simulink model "rwdEV_test01"  (R2024a)
settings: Solver=ode23t  StartTime=0.0  StopTime=2  RelTol=1e-3
model workspace (MAT data in the model file):
  f_aud = 100
libraries: fl_lib x9, sdl_lib x7, nesl_utility x6, dspsnks4 x1, ee_lib x1
settings Model: PacingRate=71  Creator=user  LastModifiedBy=user

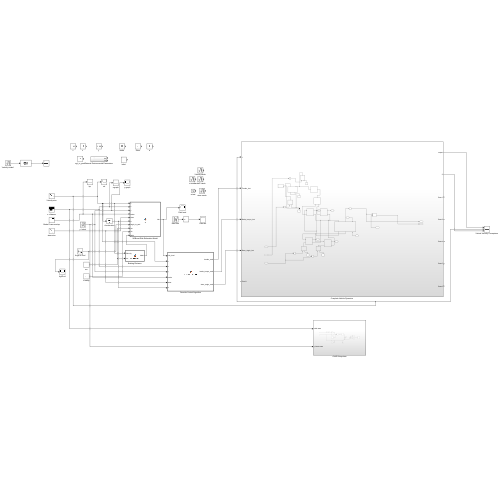
[thumbnail: Simulink's stored preview of the top-level diagram]
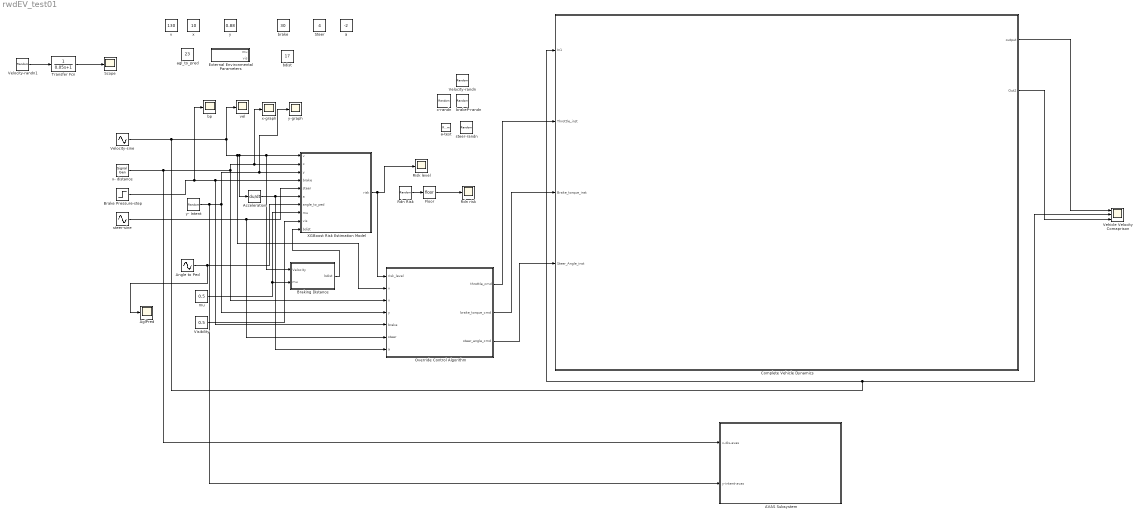
== system rwdEV_test01 ==
  AVAS Subsystem : Subsystem
  Acceleration : Derivative
  AglPred : Scope
  Angle to Ped : Sin  Amplitude=3  Frequency=0.15  SampleTime=0
  Brake Pressure-step : Step  Time=4  Before=0.2  After=0.6  SampleTime=0
  Braking Distance : MATLAB Function  TreatAsAtomicUnit=on
  "Complete Vehicle Dynamics " : Subsystem
  External Environmental Parameters : Subsystem
  Floor : Rounding
  Override Control Algorithm : MATLAB Function  TreatAsAtomicUnit=on
  Rdn Risk : UniformRandomNumber  Minimum=0  Maximum=3  SampleTime=1
  Rdn risk : Scope
  Risk level : Scope
  Scope : Scope
  Steer : Constant  Value=4
  Transfer Fcn : TransferFcn  Denominator=[0.05 1]
  Vehicle Velocity Comaprison : Scope  NumInputPorts=3
  Velocity-randn : RandomNumber  Mean=10  Variance=6  SampleTime=0.1
  Velocity-randn1 : RandomNumber  Mean=10  Variance=6  SampleTime=0.1
  Velocity-sine : Sin  Amplitude=30  Bias=180  Frequency=0.05  SampleTime=0
  Visibility : Constant  Value=0.5
  XGBoost Risk Estimation Model : MATLAB Function  TreatAsAtomicUnit=on
  a : Constant  Value=-2
  a-test : RandomNumber  Mean=3  Variance=2  SampleTime=0.1
  agl_to_pred : Constant  Value=23
  bdist : Constant  Value=17
  bp : Scope
  brake : Constant  Value=30
  brakeP-randn : RandomNumber  Mean=500  Variance=400  SampleTime=0.1
  mu : Constant  Value=0.5
  steer-randn : RandomNumber  Variance=15  SampleTime=0.1
  steer-sine : Sin  Amplitude=2  Bias=5  Frequency=0.2  SampleTime=0
  v : Constant  Value=130
  vel : Scope
  x : Constant  Value=10
  x- distance : SignalGenerator  WaveForm=random  Amplitude=0.1  Frequency=0.3  Units=rad/sec
  x-graph : Scope
  x-randn : RandomNumber  Mean=12  Variance=15  SampleTime=0.1
  y : Constant  Value=0.88
  y- Intent : RandomNumber  Mean=0.2  Variance=0.01  Seed=42  SampleTime=0.1
  y-graph : Scope
  wires:
  XGBoost Risk Estimation Model/1(risk) -> Risk level/1, Override Control Algorithm/1(risk_level)
  y- Intent/1 -> AVAS Subsystem/2(y-intent-avas), y-graph/1, XGBoost Risk Estimation Model/3(y), Override Control Algorithm/4(y)
  mu/1 -> Braking Distance/2(mu), XGBoost Risk Estimation Model/8(mu)
  Visibility/1 -> XGBoost Risk Estimation Model/9(vis)
  Braking Distance/1(bdist) -> XGBoost Risk Estimation Model/10(bdist)
  Angle to Ped/1 -> AglPred/1, XGBoost Risk Estimation Model/7(angle_to_ped)
  Velocity-sine/1 -> Vehicle Velocity Comaprison/2, "Complete Vehicle Dynamics "/1(In1), Override Control Algorithm/2(v), Braking Distance/1(Velocity), XGBoost Risk Estimation Model/1(v), Acceleration/1, vel/1
  x- distance/1 -> AVAS Subsystem/1(x-dis-avas), x-graph/1, XGBoost Risk Estimation Model/2(x), Override Control Algorithm/3(x)
  Brake Pressure-step/1 -> Override Control Algorithm/5(brake), XGBoost Risk Estimation Model/4(brake), bp/1
  steer-sine/1 -> Override Control Algorithm/6(steer), XGBoost Risk Estimation Model/5(steer)
  Acceleration/1 -> Override Control Algorithm/7(a), XGBoost Risk Estimation Model/6(a)
  Velocity-randn1/1 -> Transfer Fcn/1
  Transfer Fcn/1 -> Scope/1
  Rdn Risk/1 -> Floor/1
  Floor/1 -> Rdn risk/1
  Override Control Algorithm/1(throttle_cmd) -> "Complete Vehicle Dynamics "/2(Throttle_inst)
  Override Control Algorithm/2(brake_torque_cmd) -> "Complete Vehicle Dynamics "/3(Brake_torque_inst)
  Override Control Algorithm/3(steer_angle_cmd) -> "Complete Vehicle Dynamics "/4(Steer_Angle_inst)
  "Complete Vehicle Dynamics "/1(output) -> Vehicle Velocity Comaprison/1
  "Complete Vehicle Dynamics "/2(Out2) -> Vehicle Velocity Comaprison/3

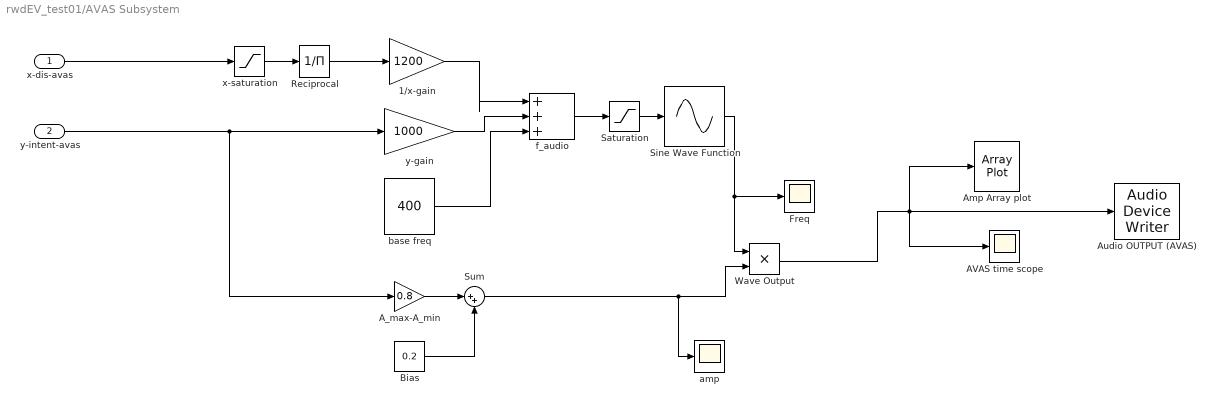
== system rwdEV_test01/AVAS Subsystem ==
  x-dis-avas : Inport
  y-intent-avas : Inport  Port=2
  1/x-gain : Gain  Gain=1200
  AVAS time scope : Scope
  A_max-A_min : Gain  Gain=0.8
  "Amp Array plot " : ArrayPlot  WindowPosition=[309.000000,216.000000,623.000000,496.000000,]  Visible=on  ScopeFrameLocation=window  YLimits=[0.02 0.0257]
  Audio OUTPUT (AVAS) : dspsnks4/Audio Device Writer  Driver=DirectSound  Device=Speaker (Realtek(R) Audio)  InheritSampleRate=off  SampleRate=44100  BitDepth=16-bit integer  BufferSize=4096  NumBuffers=10  DefaultOutputChannelMapping=on  OutputChannelMapping=1:2  OutputNumUnderrunSamples=off  DriverIdx=1  DeviceWarnFlag=''
  Bias : Constant  Value=0.2
  Freq : Scope
  Reciprocal : Product  Inputs=/
  Saturation : Saturate  UpperLimit=2500  LowerLimit=400
  Sine Wave Function : Sin  TimeSource=Use external signal  Frequency=1/44100  SampleTime=0
  Sum : Sum  Inputs=|++
  Wave Output : Product
  amp : Scope
  base freq : Constant  Value=400
  f_audio : Sum  Inputs=|+++
  x-saturation : Saturate  UpperLimit=200  LowerLimit=0.1
  y-gain : Gain  Gain=1000
  wires:
  1/x-gain/1 -> f_audio/1
  f_audio/1 -> Saturation/1
  Sine Wave Function/1 -> Wave Output/1, Freq/1
  x-saturation/1 -> Reciprocal/1
  Reciprocal/1 -> 1/x-gain/1
  base freq/1 -> f_audio/3
  y-intent-avas/1 -> A_max-A_min/1, y-gain/1
  y-gain/1 -> f_audio/2
  x-dis-avas/1 -> x-saturation/1
  Sum/1 -> amp/1, Wave Output/2
  Saturation/1 -> Sine Wave Function/1
  A_max-A_min/1 -> Sum/1
  Wave Output/1 -> AVAS time scope/1, Audio OUTPUT (AVAS)/1, "Amp Array plot "/1
  Bias/1 -> Sum/2

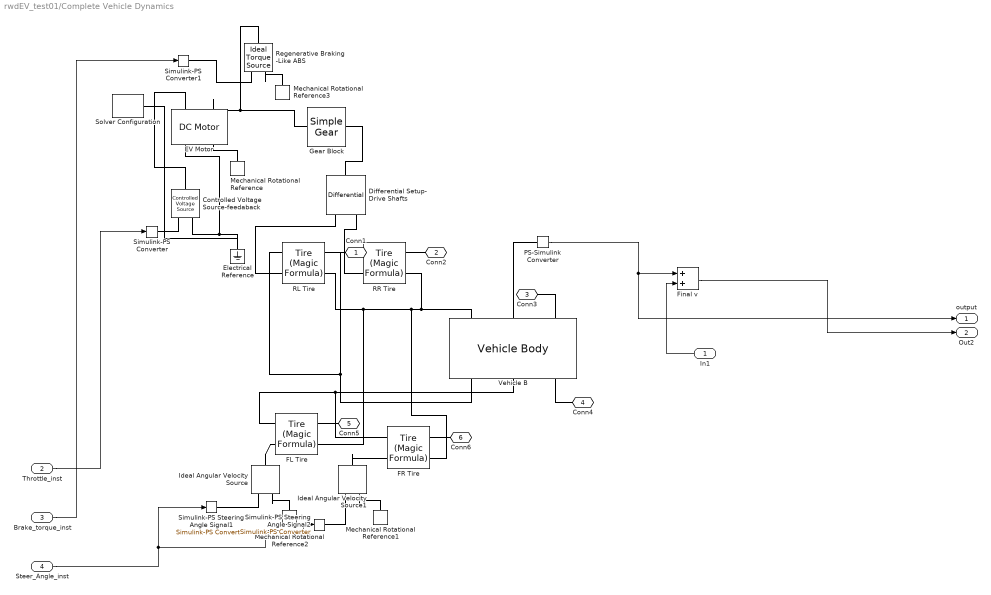
== system rwdEV_test01/Complete Vehicle Dynamics  ==
  In1 : Inport
  Throttle_inst : Inport  Port=2
  Brake_torque_inst : Inport  Port=3
  Steer_Angle_inst : Inport  Port=4
  Controlled Voltage Source-feedaback : fl_lib/Electrical/Electrical Sources/Controlled Voltage Source
  Differential Setup- Drive Shafts : sdl_lib/Gears/Differential  driveshaft_location=sdl.enum.differential_orientation.right  cd_ratio=4  friction_model=sdl.enum.gear_friction.none  efficiency=[.85, .92]  temperature_TLU=[280, 300, 320] K  efficiency_ss_TLU=[.95, .9, .85]  efficiency_cd_TLU=[.95, .9, .85]  pwr_thr=[.001, .001] W  mu_visc=[0, 0] N*m*s/rad  model_inertia=simscape.enum.onoff.off  carrier_inertia=0.001 kg*m^2  planet_inertia=0.001 kg*m^2  thermal_mass=50 J/K  T_init=300 K
  EV Motor : ee_lib/Electromechanical/Brushed Motors/DC Motor  field_option=ee.enum.field_option.pm  Rf=100 Ohm  Lf=1 H  Laf=0.15 H  If0=0 A  parameterization=ee.enum.dcparam_option.circuit_param  Ra=3.9 Ohm  La=12e-6 H  emf_or_torque=ee.enum.emf_or_torque.kv  Kv=0.072e-3 V/rpm  Ki=6.876e-4 N*m/A  T_stall=0.24e-3 N*m  w_max=19100 rpm  w_rated=15000 rpm  P_rated=0.08 W  V_rated=1.5 V  lam_param=ee.enum.lam_param.damping  i_noload=0 A  V_i_noload=1.5 V  J=0.01 cm^2*g  lam=0 N*m*s/rad  speed0=0 rpm  enable_fault_armature=simscape.enum.onoff.off  rev_faulted=1 / 3  G_faulted_armature=1e-5 S  fault_trigger_armature=ee.enum.faults.faultTrigger.temporal  t_fault_armature=1 s  max_permissible_current_armature=inf A  t_fail_on_current_armature=1 s  enable_fault_field=simscape.enum.onoff.off  G_faulted_field=1e-5 S  fault_trigger_field=ee.enum.faults.faultTrigger.temporal  t_fault_field=1 s  max_permissible_current_field=inf A  t_fail_on_current_field=1 s  fault_action=simscape.enum.assert.action.none  alpha=3.93e-3 1/K  Tmeas=25 degC  thermal_mass=100 J/K  initial_temperature=25 degC
  Electrical Reference : fl_lib/Electrical/Electrical Elements/Electrical Reference
  FL Tire : sdl_lib/Tires & Vehicles/Tire (Magic Formula)  parameterization=sdl.enum.magic_tire_model.peak  F_z1=3000 N  F_x1=3500 N  kappa1=10  B_m=10  C_m=1.9  D_m=1  E_m=0.97  fz0=4000 N  p_Cx=1.685  p_Dx=[1.21, -.037]  p_Ex=[.344, .095, -.02, 0]  p_Kx=[21.51, -.163, .245]  p_Hx=[-.002, .002]  p_Vx=[0, 0]  rolling_radius_model=sdl.enum.RollingRadiusParameterization.Constant  r_e=0.3 m  r_0=0.3 m  breff=8.39  dreff=0.26  freff=0.074  q_re0=0.99  q_v1=0.008  longvl=17 m/s  cz=5e5 N/m  model_resistance=false  resistance_model=sdl.enum.rollingResistanceParameterization.constant  coeff=0.015  p_tire=250e3 Pa  alpha=-0.003  beta=0.97  coeff_a=84e-4  coeff_b=6.2e-4 s/m  coeff_c=1.6e-4 s^2/m^2  p_tire0=240e3 Pa  fz0_resistance=4000 N  vH0=16 m/s  q_Sy=[.0082, 0, .0014, .001, 0, 0, 1.08, -.5]  v_thr=0.001 m/s  enable_scaling_coefficients=false  lfzO=1  lcx=1  lmux=1  lex=1  lkx=1  lhx=1  lvx=1  lmy=1  model_compliance=sdl.enum.compliance.off  stiffness=1e6 N/m  damping=1000 N*s/m  model_inertia=sdl.enum.model_inertia.off  inertia=1 kg*m^2  initial_velocity=0 rad/s  vxlow=1 m/s  v_tr_thr=0.1 m/s  kpumin=-1.5  kpumax=1.5
  FR Tire : sdl_lib/Tires & Vehicles/Tire (Magic Formula)  parameterization=sdl.enum.magic_tire_model.peak  F_z1=3000 N  F_x1=3500 N  kappa1=10  B_m=10  C_m=1.9  D_m=1  E_m=0.97  fz0=4000 N  p_Cx=1.685  p_Dx=[1.21, -.037]  p_Ex=[.344, .095, -.02, 0]  p_Kx=[21.51, -.163, .245]  p_Hx=[-.002, .002]  p_Vx=[0, 0]  rolling_radius_model=sdl.enum.RollingRadiusParameterization.Constant  r_e=0.3 m  r_0=0.3 m  breff=8.39  dreff=0.26  freff=0.074  q_re0=0.99  q_v1=0.008  longvl=17 m/s  cz=5e5 N/m  model_resistance=false  resistance_model=sdl.enum.rollingResistanceParameterization.constant  coeff=0.015  p_tire=250e3 Pa  alpha=-0.003  beta=0.97  coeff_a=84e-4  coeff_b=6.2e-4 s/m  coeff_c=1.6e-4 s^2/m^2  p_tire0=240e3 Pa  fz0_resistance=4000 N  vH0=16 m/s  q_Sy=[.0082, 0, .0014, .001, 0, 0, 1.08, -.5]  v_thr=0.001 m/s  enable_scaling_coefficients=false  lfzO=1  lcx=1  lmux=1  lex=1  lkx=1  lhx=1  lvx=1  lmy=1  model_compliance=sdl.enum.compliance.off  stiffness=1e6 N/m  damping=1000 N*s/m  model_inertia=sdl.enum.model_inertia.off  inertia=1 kg*m^2  initial_velocity=0 rad/s  vxlow=1 m/s  v_tr_thr=0.1 m/s  kpumin=-1.5  kpumax=1.5
  Final v : Sum
  Gear Block : sdl_lib/Gears/Simple Gear  ratio=2  rotation_direction=sdl.enum.shaftOutputDirection.opposite  enable_faults=simscape.enum.onoff.off  efficiency_fault=0.05  fault_angles=pi / 12 rad  friction_model=sdl.enum.gear_efficiencies_load.off  T_noload=0.1 N*m  T_nom=5 N*m  efficiency_nom=0.8  efficiency=0.8  temperature_TLU=[280, 300, 320] K  load_TLU=[1, 5, 10] N*m  efficiency_TLU=[.95, .9, .85]  efficiency_TLU2=[.85, .8, .75; .95, .9, .85; .85, .8, .7]  w_thr=0.01 rad/s  pwr_thr=0.001 W  enable_backlash=false  hardstop_model=simscape.enum.hardstop.smooth  backlash_distance=1e-3 mm  r_base=0.1 m  transition=1e-4 mm  backlash_stiffness=1e6 N/m  backlash_damping=1e3 N*s/m  coeff_rest=0.7  v_tol=0.001 m/s  f_tol=0.001 N  mu_visc=[0, 0] N*m*s/rad  thermal_mass=50 J/K  temperature_specify=off  temperature_priority=High  temperature=300 K  temperature_nominal_specify=off  temperature_nominal_value=1  temperature_nominal_unit=K  x_backlash_specify=off  x_backlash_priority=None  x_backlash=0 mm  x_backlash_nominal_specify=off  x_backlash_nominal_value=1  x_backlash_nominal_unit=mm  f_hardstop_specify=off  f_hardstop_priority=None  f_hardstop=0 N  f_hardstop_nominal_specify=off  f_hardstop_nominal_value=1  f_hardstop_nominal_unit=N  v_backlash_specify=off  v_backlash_priority=None  v_backlash=0 m/s  v_backlash_nominal_specify=off  v_backlash_nominal_value=1  v_backlash_nominal_unit=m/s
  Ideal Angular Velocity Source : fl_lib/Mechanical/Mechanical Sources/Ideal Angular Velocity Source
  Ideal Angular Velocity Source1 : fl_lib/Mechanical/Mechanical Sources/Ideal Angular Velocity Source
  Mechanical Rotational Reference{,1..3} (4 alike) : fl_lib/Mechanical/Rotational Elements/Mechanical Rotational Reference
  PS-Simulink Converter : nesl_utility/PS-Simulink Converter  PhysicalDomain=network_engine_domain  SubClassName=ps_output  LeftPortType=input  RightPortType=output  PseudoPeriodic=off  Frequencies=[]  VectorFormat=inherit  Unit=m/s  AffineConversion=off
  RL Tire : sdl_lib/Tires & Vehicles/Tire (Magic Formula)  parameterization=sdl.enum.magic_tire_model.peak  F_z1=3000 N  F_x1=3500 N  kappa1=10  B_m=10  C_m=1.9  D_m=1  E_m=0.97  fz0=4000 N  p_Cx=1.685  p_Dx=[1.21, -.037]  p_Ex=[.344, .095, -.02, 0]  p_Kx=[21.51, -.163, .245]  p_Hx=[-.002, .002]  p_Vx=[0, 0]  rolling_radius_model=sdl.enum.RollingRadiusParameterization.Constant  r_e=0.3 m  r_0=0.3 m  breff=8.39  dreff=0.26  freff=0.074  q_re0=0.99  q_v1=0.008  longvl=17 m/s  cz=5e5 N/m  model_resistance=false  resistance_model=sdl.enum.rollingResistanceParameterization.constant  coeff=0.015  p_tire=250e3 Pa  alpha=-0.003  beta=0.97  coeff_a=84e-4  coeff_b=6.2e-4 s/m  coeff_c=1.6e-4 s^2/m^2  p_tire0=240e3 Pa  fz0_resistance=4000 N  vH0=16 m/s  q_Sy=[.0082, 0, .0014, .001, 0, 0, 1.08, -.5]  v_thr=0.001 m/s  enable_scaling_coefficients=false  lfzO=1  lcx=1  lmux=1  lex=1  lkx=1  lhx=1  lvx=1  lmy=1  model_compliance=sdl.enum.compliance.off  stiffness=1e6 N/m  damping=1000 N*s/m  model_inertia=sdl.enum.model_inertia.off  inertia=1 kg*m^2  initial_velocity=0 rad/s  vxlow=1 m/s  v_tr_thr=0.1 m/s  kpumin=-1.5  kpumax=1.5
  RR Tire : sdl_lib/Tires & Vehicles/Tire (Magic Formula)  parameterization=sdl.enum.magic_tire_model.peak  F_z1=3000 N  F_x1=3500 N  kappa1=10  B_m=10  C_m=1.9  D_m=1  E_m=0.97  fz0=4000 N  p_Cx=1.685  p_Dx=[1.21, -.037]  p_Ex=[.344, .095, -.02, 0]  p_Kx=[21.51, -.163, .245]  p_Hx=[-.002, .002]  p_Vx=[0, 0]  rolling_radius_model=sdl.enum.RollingRadiusParameterization.Constant  r_e=0.3 m  r_0=0.3 m  breff=8.39  dreff=0.26  freff=0.074  q_re0=0.99  q_v1=0.008  longvl=17 m/s  cz=5e5 N/m  model_resistance=false  resistance_model=sdl.enum.rollingResistanceParameterization.constant  coeff=0.015  p_tire=250e3 Pa  alpha=-0.003  beta=0.97  coeff_a=84e-4  coeff_b=6.2e-4 s/m  coeff_c=1.6e-4 s^2/m^2  p_tire0=240e3 Pa  fz0_resistance=4000 N  vH0=16 m/s  q_Sy=[.0082, 0, .0014, .001, 0, 0, 1.08, -.5]  v_thr=0.001 m/s  enable_scaling_coefficients=false  lfzO=1  lcx=1  lmux=1  lex=1  lkx=1  lhx=1  lvx=1  lmy=1  model_compliance=sdl.enum.compliance.off  stiffness=1e6 N/m  damping=1000 N*s/m  model_inertia=sdl.enum.model_inertia.off  inertia=1 kg*m^2  initial_velocity=0 rad/s  vxlow=1 m/s  v_tr_thr=0.1 m/s  kpumin=-1.5  kpumax=1.5
  Regenerative Braking -Like ABS : fl_lib/Mechanical/Mechanical Sources/Ideal Torque Source
  Simulink-PS Converter : nesl_utility/Simulink-PS Converter  PhysicalDomain=network_engine_domain  SubClassName=ps_input  LeftPortType=input  RightPortType=output  PseudoPeriodic=off  Frequencies=[]  NoiseDistribution=none  NoiseParameters=[]  Unit=V  AffineConversion=off  FilteringAndDerivatives=provide  SimscapeFilterOrder=1  InputFilterTimeConstant=0.001  UdotUserProvided=0
  Simulink-PS Converter1 : nesl_utility/Simulink-PS Converter  PhysicalDomain=network_engine_domain  SubClassName=ps_input  LeftPortType=input  RightPortType=output  PseudoPeriodic=off  Frequencies=[]  NoiseDistribution=none  NoiseParameters=[]  Unit=N*m  AffineConversion=off  FilteringAndDerivatives=provide  SimscapeFilterOrder=1  InputFilterTimeConstant=0.001  UdotUserProvided=0
  Simulink-PS Steering Angle Signal1 : nesl_utility/Simulink-PS Converter  PhysicalDomain=network_engine_domain  SubClassName=ps_input  LeftPortType=input  RightPortType=output  PseudoPeriodic=off  Frequencies=[]  NoiseDistribution=none  NoiseParameters=[]  Unit=rad/s  AffineConversion=off  FilteringAndDerivatives=provide  SimscapeFilterOrder=1  InputFilterTimeConstant=0.001  UdotUserProvided=0
  Simulink-PS Steering Angle Signal2 : nesl_utility/Simulink-PS Converter  PhysicalDomain=network_engine_domain  SubClassName=ps_input  LeftPortType=input  RightPortType=output  PseudoPeriodic=off  Frequencies=[]  NoiseDistribution=none  NoiseParameters=[]  Unit=rad/s  AffineConversion=off  FilteringAndDerivatives=provide  SimscapeFilterOrder=1  InputFilterTimeConstant=0.001  UdotUserProvided=0
  Solver Configuration : nesl_utility/Solver Configuration  PhysicalDomain=network_engine_domain  SubClassName=solver  LeftPortType=input  RightPortType=generic  Tones=[]  Harmonics=[]  SimulateNoise=off  Profile=off  UseLocalSampling=off  EnableSwitchedLinearOptims=on  FrequencyDomain=off  UseCCode=off  RelTol=0.001  AbsTol=0.001  MinStep=1e-09  ToWorkspace=off  RevertToSquareIcSolve=off  NumHomotopyIterations=100  PhasorMode=off  PhasorModeNumHarmonics=1  ConsistencySolver=NEWTON_XTOL_AFTER_FTOL  IndexReductionMethod=DerivativeReplacement  DoDC=off  ResidualTolerance=1e-09  ConsistencyTolSource=GLOBAL  ConsistencyAbsTol=0.001  ConsistencyRelTol=0.001  ConsistencyTolFactor=0.001  UseLocalSolver=off  LocalSolverChoice=NE_BACKWARD_EULER_ADVANCER  ResolveIndetEquations=on  FunctionEvalNumThread=1  LocalSolverSampleTime=0.001  DoFixedCost=off  MaxNonlinIter=3  MaxModeIter=2  ComputeImpulses=off  ImpulseIterations=2  LinearAlgebra=auto  LinearAlgebraNumThread=0  EquationFormulation=NE_TIME_EF  DelaysMemoryBudget=1024  AutomaticFiltering=on  FilteringTimeConstant=0.001  PartitionStorageMethod=AS_NEEDED  PartitionMemoryBudget=1024  PartitionMethod=ROBUST  MultibodyUseLocalSolver=off  MultibodyLocalSolverChoice=ODE1  MultibodyLocalSolverSampleTime=0.001
  Vehicle B : sdl_lib/Tires & Vehicles/Vehicle Body  mass=1200 kg  n_w=2  x_f=1.4 m  x_r=1.6 m  y_c=0.5 m  mass_var=simscape.enum.onoff.off  g=9.81 m/s^2  liftoff_warning=simscape.enum.onoff.off  area=3 m^2  Cd=0.4  rho=1.18 kg/m^3  model_pitch=simscape.enum.onoff.off  inertia=4000 kg*m^2  suspension_model=sdl.enum.linearTLU.linear  k_f=1e4 N/m  b_f=1e4 N*s/m  k_r=1e4 N/m  b_r=1e4 N*s/m  k_f_TLU=[-2000, -1000, 0, 1000, 2000] N  x_f_TLU=[-.4, -.2, 0, .2, .4] m  b_f_TLU=[-200, -100, 0, 100, 200] N  v_f_TLU=[-4, -2, 0, 2, 4] m/s  k_r_TLU=[-2000, -1000, 0, 1000, 2000] N  x_r_TLU=[-.4, -.2, 0, .2, .4] m  b_r_TLU=[-200, -100, 0, 100, 200] N  v_r_TLU=[-4, -2, 0, 2, 4] m/s  interp_method=simscape.enum.interpolation.linear  extrap_method=simscape.enum.extrapolation.linear  model_hardstop=simscape.enum.onoff.off  upper_bound_f=.25 m  lower_bound_f=-.25 m  stop_k_f=1e6 N/m  stop_b_f=150 N*s/m  upper_bound_r=.25 m  lower_bound_r=-.25 m  stop_k_r=1e6 N/m  stop_b_r=150 N*s/m  initial_pitch=0 rad  initial_pitch_rate=0 rad/s  v_specify=off  v_priority=High  v=0 m/s  v_nominal_specify=off  v_nominal_value=1  v_nominal_unit=m/s
  Conn1 : PMIOPort  Side=Right
  Conn2 : PMIOPort  Port=2  Side=Right
  Conn3 : PMIOPort  Port=3  Side=Left
  Conn4 : PMIOPort  Port=4  Side=Right
  Conn5 : PMIOPort  Port=5  Side=Right
  Conn6 : PMIOPort  Port=6  Side=Right
  output : Outport
  Out2 : Outport  Port=2
  wires:
  Brake_torque_inst/1 -> Simulink-PS Converter1/1
  PS-Simulink Converter/1 -> output/1, Final v/1
  Throttle_inst/1 -> Simulink-PS Converter/1
  Final v/1 -> Out2/1
  Steer_Angle_inst/1 -> Simulink-PS Steering Angle Signal1/1, Simulink-PS Steering Angle Signal2/1
  In1/1 -> Final v/2
  connections:
  FR Tire/RConn1 -- Conn6/RConn1
  Controlled Voltage Source-feedaback/LConn1 -- EV Motor/LConn1
  RL Tire/RConn2 -- FL Tire/RConn2 -- FR Tire/RConn2 -- RR Tire/RConn2 -- Vehicle B/LConn1
  Controlled Voltage Source-feedaback/RConn2 -- Solver Configuration/RConn1 -- Electrical Reference/LConn1 -- EV Motor/RConn1
  Mechanical Rotational Reference/LConn1 -- EV Motor/RConn2
  RR Tire/LConn1 -- RL Tire/LConn1 -- Vehicle B/RConn1
  Gear Block/RConn1 -- Differential Setup- Drive Shafts/LConn1
  Ideal Angular Velocity Source1/LConn1 -- FR Tire/LConn2
  Differential Setup- Drive Shafts/RConn1 -- RL Tire/LConn2
  Simulink-PS Converter/RConn1 -- Controlled Voltage Source-feedaback/RConn1
  Differential Setup- Drive Shafts/RConn2 -- RR Tire/LConn2
  EV Motor/LConn2 -- Regenerative Braking -Like ABS/LConn1 -- Gear Block/LConn1
  Simulink-PS Steering Angle Signal2/RConn1 -- Ideal Angular Velocity Source1/RConn1
  Vehicle B/RConn2 -- FR Tire/LConn1 -- FL Tire/LConn1
  Simulink-PS Steering Angle Signal1/RConn1 -- Ideal Angular Velocity Source/RConn1
  Regenerative Braking -Like ABS/RConn2 -- Mechanical Rotational Reference3/LConn1
  Ideal Angular Velocity Source/LConn1 -- FL Tire/LConn2
  Vehicle B/RConn3 -- Conn4/RConn1
  Ideal Angular Velocity Source1/RConn2 -- Mechanical Rotational Reference1/LConn1
  Ideal Angular Velocity Source/RConn2 -- Mechanical Rotational Reference2/LConn1
  Vehicle B/LConn2 -- PS-Simulink Converter/LConn1
  RL Tire/RConn1 -- Conn1/RConn1
  Simulink-PS Converter1/RConn1 -- Regenerative Braking -Like ABS/RConn1
  FL Tire/RConn1 -- Conn5/RConn1
  RR Tire/RConn1 -- Conn2/RConn1
  Vehicle B/LConn3 -- Conn3/RConn1

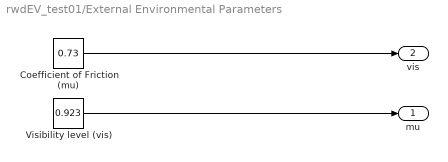
== system rwdEV_test01/External Environmental Parameters ==
  Coefficient of Friction (mu) : Constant  Value=0.73
  Visibility level (vis) : Constant  Value=0.923
  mu : Outport
  vis : Outport  Port=2
  wires:
  Visibility level (vis)/1 -> mu/1
  Coefficient of Friction (mu)/1 -> vis/1

== matlab function rwdEV_test01/XGBoost Risk Estimation Model ==
  data: v input; risk output; x input; y input; brake input; steer input; a input; angle_to_ped input; mu input; vis input; bdist input

% function risk_level = xgb(v, x, y, brake, steer, a, angle_to_ped, mu, vis, bdist)
% %#codegen
% 
%     % Declare Python-callable function
%     coder.extrinsic('xgb_predict');
% 
%     % Input vector of all parameters
%     input_vector = [v, x, y, brake, steer, a, angle_to_ped, mu, vis, bdist];
% 
%     % Initialize
%     risk_level = int32(0);  % default risk level
% 
%     % Call Python-side function (defined below)
%     risk_py = xgb_predict(input_vector);
% 
%     if ~isempty(risk_py)
%         risk_level = int32(risk_py);
%     end
% end

function risk = fcn(v, x, y, brake, steer, a, angle_to_ped, mu, vis, bdist)
    %#codegen

    % Initialize output
    risk = int32(0);

    % Mark as external
    coder.extrinsic('xgb_predict_new');

    % Form input vector
    input_vec = [v, x, y, brake, steer, a, angle_to_ped, mu, vis, bdist];

    % Call Python-based predictor
    risk_pred = xgb_predict_new(input_vec);

    % Assign to output
    if ~isempty(risk_pred)
        risk = int32(risk_pred);
    end
end

== matlab function rwdEV_test01/Override Control Algorithm ==
  data: risk_level input; throttle_cmd output; brake_torque_cmd output; steer_angle_cmd output; v input; x input; y input; brake input; steer input; a input
% function [throttle_cmd, brake_torque_cmd, steer_angle_cmd] = override_control(risk_level, v, x, y, brake, steer, a)
% %#codegen
% % Inputs:
% %   risk_level        : int (0=A1, 1=A2, 2=A3)
% %   v                 : vehicle speed (m/s)
% %   x                 : pedestrian distance ahead (m)
% %   y                 : pedestrian intent score (0–1)
% %   brake             : current brake torque (Nm)
% %   steer             : current steering angle (degrees)
% %   a                 : vehicle acceleration (m/s^2)
% %
% % Outputs:
% %   throttle_cmd      : 0 to 1 normalized throttle
% %   brake_torque_cmd  : Nm (0 to max_brake_torque)
% %   steer_angle_cmd   : degrees
% 
%     %% Control limits
%     max_throttle = 1.0;
%     max_brake_torque = 1500;  % Nm
%     max_steering_angle = 30;  % degrees
% 
%     %% Defaults from current state
%     throttle_cmd = a_to_throttle(a, max_throttle);
%     brake_torque_cmd = clamp(brake, 0, max_brake_torque);
%     steer_angle_cmd = clamp(steer, -max_steering_angle, max_steering_angle);
% 
%     %% Time-to-Collision (TTC)
%     v_safe = max(v, 0.1);  % avoid divide-by-zero
%     ttc = x / v_safe;
% 
%     %% Override based on risk level
%     if risk_level == 1  % A2: Medium risk – override partially
%         if ttc < 3 || y > 0.6
%             throttle_cmd = 0.2;
%             brake_torque_cmd = clamp(brake + 400, 0, max_brake_torque);
%             steer_angle_cmd = limit_steering(steer, max_steering_angle);
%         end
% 
%     elseif risk_level == 2  % A3: High risk – emergency override
%         throttle_cmd = 0.0;
%         brake_torque_cmd = max_brake_torque;
% 
%         % Evasive steering
%         if steer == 0
%             steer_angle_cmd = 15;
%         elseif steer > 0
%             steer_angle_cmd = clamp(steer + 10, 0, max_steering_angle);
%         else
%             steer_angle_cmd = clamp(steer - 10, -max_steering_angle, 0);
%         end
%     end
% end
% 
% %% Helper: Acceleration to Throttle
% function throttle = a_to_throttle(a, max_throttle)
%     throttle = clamp(a / 3.0, 0, max_throttle);  % scale factor (adjustable)
% end
% 
% %% Helper: Clamp value between min and max
% function val = clamp(val, min_val, max_val)
%     val = min(max(val, min_val), max_val);
% end
% 
% %% Helper: Limit steering angle
% function angle = limit_steering(angle, max_angle)
%     angle = clamp(angle, -max_angle, max_angle);
% end

function [throttle_cmd, brake_torque_cmd, steer_angle_cmd] = override_control(risk_level, v, x, y, brake, steer, a)
%#codegen

%% Parameters
max_throttle = 1.0;              % Full throttle
max_brake_torque = 1800;         % Nm (typical for electric braking)
max_steering_angle = 30;         % degrees
min_ttc_emergency = 1.5;         % seconds (for A3)
min_ttc_alert = 3.0;             % seconds (for A2)

% Smoother steering buffer to reduce jerks
steer_buffer = 5;

%% Default to current state
throttle_cmd = a_to_throttle(a, max_throttle);
brake_torque_cmd = clamp(brake, 0, max_brake_torque);
steer_angle_cmd = clamp(steer, -max_steering_angle, max_steering_angle);

% Calculate Time-To-Collision (TTC)
v_safe = max(v, 0.5);  % Prevent division by zero
ttc = x / v_safe;

%% A2 (Alert) Logic
if risk_level == 1
    if (ttc < min_ttc_alert || y > 0.6)
        % Slight override
        throttle_cmd = 0.3;
        brake_torque_cmd = clamp(brake + 500, 0, max_brake_torque);
        steer_angle_cmd = clamp(steer, -max_steering_angle + steer_buffer, max_steering_angle - steer_buffer);
    end

%% A3 (Emergency) Logic
elseif risk_level == 2
    if (ttc < min_ttc_emergency || y > 0.8)
        % Emergency full override
        throttle_cmd = 0.0;
        brake_torque_cmd = max_brake_torque;

        % Evasive steering based on current steer value
        if steer == 0
            steer_angle_cmd = 15;
        elseif steer > 0
            steer_angle_cmd = clamp(steer + steer_buffer, 0, max_steering_angle);
        else
            steer_angle_cmd = clamp(steer - steer_buffer, -max_steering_angle, 0);
        end
    end
end
end

%% Helper: Acceleration to Throttle Conversion
function throttle = a_to_throttle(a, max_throttle)
    throttle = clamp(0.4 + a / 4.0, 0, max_throttle);  % Slight buffer included
end

%% Helper: Clamp values
function val = clamp(val, min_val, max_val)
    val = min(max(val, min_val), max_val);
end

== matlab function rwdEV_test01/Braking Distance ==
  data: Velocity input; bdist output; mu input
function bdist = brakingDist(Velocity, mu)

bdist = (Velocity^2)/(2*mu*9.8);
